simulink model "porte_avion_echantionne_model"  (R2025b)
settings: Solver=VariableStepAuto  StartTime=0.0  StopTime=100  RelTol=1e-3
values from neighbouring files (symbols this model uses):
  Ac = [0 1 0 0 ... (first row only)    [porte_avion_ech.m]
  Ad = ssd.A    [porte_avion_ech.m]
  Bc = [0 ... (first row only)    [porte_avion_ech.m]
  Bd = ssd.B    [porte_avion_ech.m]
  Cc = [0 0 1 0]    [porte_avion_ech.m]
  Cd = ssd.C    [porte_avion_ech.m]
  Hc = -1 / (Cc * ((Ac - Bc*Kc) \ Bc))    [porte_avion_ech.m]
  Hd = 1 / (Cd * ((eye(4) - (Ad - Bd*Kd)) \ Bd))    [porte_avion_ech.m]
  Kc = place(Ac, Bc, poles_c)    [porte_avion_ech.m]
  Kd = place(Ad, Bd, poles_d)    [porte_avion_ech.m]
  Ts = Tss(3)    [porte_avion_ech.m]
  X_0 = [x_0 ... (first row only)    [porte_avion_ech.m]
undefined symbols (not defined in the file or in its folder): A, A_obs, B, B_obs, C, C_obs, D, H, K, L_obs, r
settings Model: Creator=victor  LastModifiedBy=victor

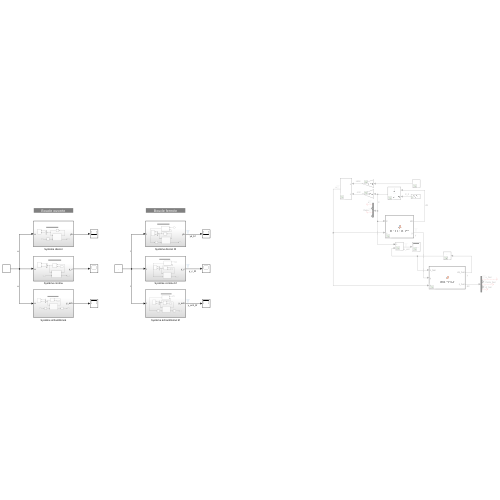
[thumbnail: Simulink's stored preview of the top-level diagram]
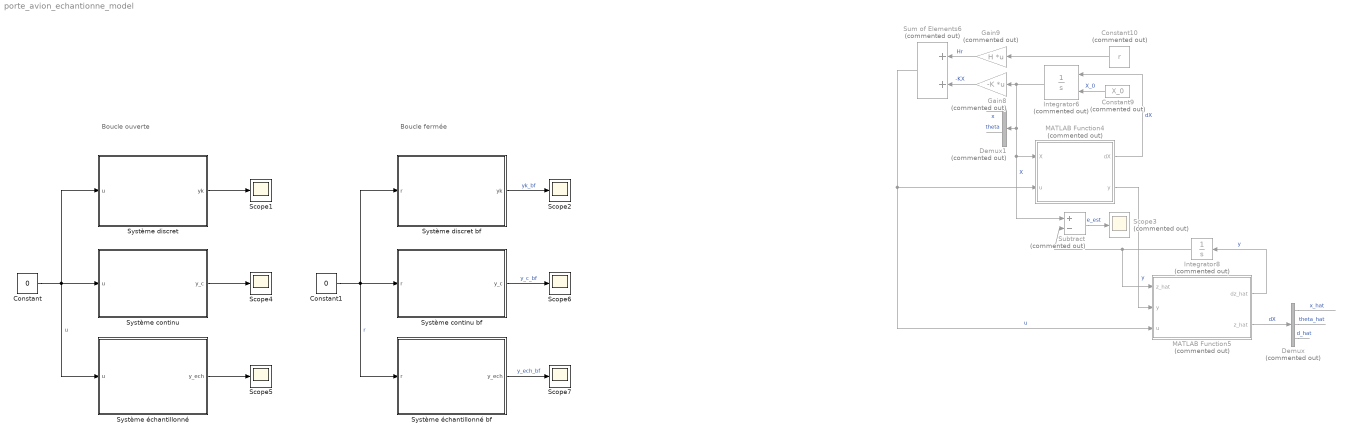
== system porte_avion_echantionne_model ==
  note: Boucle ouverte
  note: Boucle fermée
  Constant : Constant  Value=0
  Constant1 : Constant  Value=0
  Constant10 : Constant  Commented=on  Value=r
  Constant9 : Constant  Commented=on  Value=X_0
  Demux : Demux  Commented=on  Outputs=5
  Demux1 : Demux  Commented=on
  Gain8 : Gain  Commented=on  Gain=-K  Multiplication=Matrix(K*u)
  Gain9 : Gain  Commented=on  Gain=H  Multiplication=Matrix(K*u)
  Integrator6 : Integrator  Commented=on  InitialConditionSource=external
  Integrator8 : Integrator  Commented=on  InitialCondition=zeros(5, 1)
  MATLAB Function4 : MATLAB Function  Commented=on  TreatAsAtomicUnit=on
  MATLAB Function5 : MATLAB Function  Commented=on  TreatAsAtomicUnit=on
  Scope{1..2,4..7} (6 alike) : Scope
      Scope1 settings: ActiveDisplayYMinimum=-1  ActiveDisplayYMaximum=1
      Scope2 settings: ActiveDisplayYMinimum=-1  ActiveDisplayYMaximum=1  DataLoggingVariableName=ScopeData7
      Scope4 settings: ActiveDisplayYMinimum=-0.17297207419150878  ActiveDisplayYMaximum=0.36828496975347796  DataLoggingVariableName=ScopeData4
      Scope5 settings: ActiveDisplayYMinimum=-0.17297207419150878  ActiveDisplayYMaximum=0.36828496975347796  DataLoggingVariableName=ScopeData5
      Scope6 settings: ActiveDisplayYMinimum=-0.17297207419150878  ActiveDisplayYMaximum=0.36828496975347796  DataLoggingVariableName=ScopeData8
      Scope7 settings: ActiveDisplayYMinimum=-0.17297207419150878  ActiveDisplayYMaximum=0.36828496975347796  DataLoggingVariableName=ScopeData9
  Scope3 : Scope  Commented=on
      settings: ActiveDisplayYMinimum=-1.369875447599938  ActiveDisplayYMaximum=0.62027967456851218  DataLoggingVariableName=ScopeData3
  Subtract : Sum  Commented=on  Inputs=+-
  Sum of Elements6 : Sum  Commented=on
  Système continu : Subsystem
  Système continu bf : Subsystem
  Système discret : Subsystem
  Système discret bf : Subsystem
  Système échantillonné : Subsystem
  Système échantillonné bf : Subsystem
  wires:
  Demux/1 -> ?  "x_hat"
  Gain8/1 -> Sum of Elements6/2  "-KX"
  Demux/5 -> ?  "d_hat"
  Demux1/3 -> ?  "theta"
  MATLAB Function5/1(dz_hat) -> Integrator8/1  "y"
  Sum of Elements6/1 -> MATLAB Function4/2(u), MATLAB Function5/3(u)  "u"
  Demux/3 -> ?  "theta_hat"
  Integrator8/1 -> MATLAB Function5/1("z_hat "), Subtract/2
  Demux1/1 -> ?  "x"
  MATLAB Function4/2(y) -> MATLAB Function5/2(y)  "y"
  Gain9/1 -> Sum of Elements6/1  "Hr"
  MATLAB Function4/1(dX) -> Integrator6/1  "dX"
  MATLAB Function5/2(z_hat) -> Demux/1  "dX"
  Constant10/1 -> Gain9/1
  Subtract/1 -> Scope3/1  "e_est"
  Integrator6/1 -> Subtract/1, MATLAB Function4/1(X), Demux1/1, Gain8/1  "X"
  Constant9/1 -> Integrator6/2  "X_0"
  Constant/1 -> Système échantillonné/1(u), Système discret/1(u), Système continu/1(u)  "u"
  Système discret/1(yk) -> Scope1/1
  Système continu/1(y_c) -> Scope4/1
  Système échantillonné/1(y_ech) -> Scope5/1
  Système discret bf/1(yk) -> Scope2/1  "yk_bf"
  Constant1/1 -> Système échantillonné bf/1(r), Système discret bf/1(r), Système continu bf/1(r)  "r"
  Système continu bf/1(y_c) -> Scope6/1  "y_c_bf"
  Système échantillonné bf/1(y_ech) -> Scope7/1  "y_ech_bf"

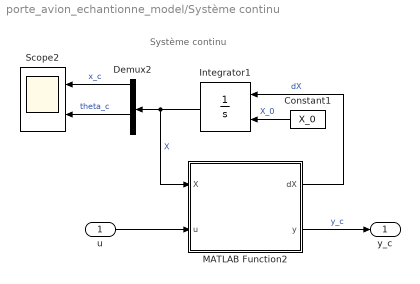
== system porte_avion_echantionne_model/Système continu ==
  note: Système continu
  u : Inport
  Constant1 : Constant  Value=X_0
  Demux2 : Demux
  Integrator1 : Integrator  InitialConditionSource=external
  MATLAB Function2 : MATLAB Function  TreatAsAtomicUnit=on
  Scope2 : Scope  NumInputPorts=2
      settings: ActiveDisplayYMinimum=-33.650451529708675  ActiveDisplayYMaximum=4.0880049092553845  DataLoggingVariableName=ScopeData2
  y_c : Outport
  wires:
  Integrator1/1 -> MATLAB Function2/1(X), Demux2/1  "X"
  Demux2/1 -> Scope2/1  "x_c"
  Demux2/3 -> Scope2/2  "theta_c"
  Constant1/1 -> Integrator1/2  "X_0"
  u/1 -> MATLAB Function2/2(u)
  MATLAB Function2/1(dX) -> Integrator1/1  "dX"
  MATLAB Function2/2(y) -> y_c/1  "y_c"

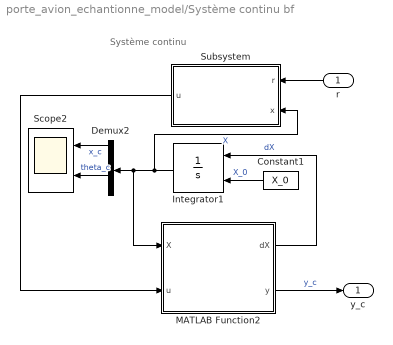
== system porte_avion_echantionne_model/Système continu bf ==
  note: Système continu
  r : Inport
  Constant1 : Constant  Value=X_0
  Demux2 : Demux
  Integrator1 : Integrator  InitialConditionSource=external
  MATLAB Function2 : MATLAB Function  TreatAsAtomicUnit=on
  Scope2 : Scope  NumInputPorts=2
      settings: ActiveDisplayYMinimum=-33.650451529708675  ActiveDisplayYMaximum=4.0880049092553845  DataLoggingVariableName=ScopeData2
  Subsystem : Subsystem
  y_c : Outport
  wires:
  Integrator1/1 -> Subsystem/2(x), MATLAB Function2/1(X), Demux2/1  "X"
  Demux2/1 -> Scope2/1  "x_c"
  Demux2/3 -> Scope2/2  "theta_c"
  Constant1/1 -> Integrator1/2  "X_0"
  Subsystem/1(u) -> MATLAB Function2/2(u)
  MATLAB Function2/1(dX) -> Integrator1/1  "dX"
  MATLAB Function2/2(y) -> y_c/1  "y_c"
  r/1 -> Subsystem/1(r)

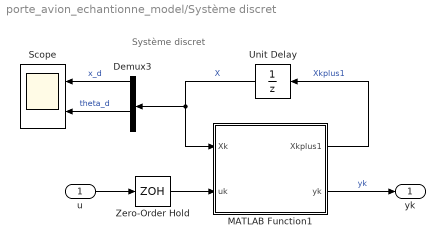
== system porte_avion_echantionne_model/Système discret ==
  note: Système discret
  u : Inport
  Demux3 : Demux
  MATLAB Function1 : MATLAB Function  TreatAsAtomicUnit=on  SystemSampleTime=Ts
  Scope : Scope  NumInputPorts=2
      settings: ActiveDisplayYMinimum=-1  ActiveDisplayYMaximum=1
  Unit Delay : UnitDelay  InitialCondition=X_0  SampleTime=-1  HasFrameUpgradeWarning=on
  Zero-Order Hold : ZeroOrderHold  SampleTime=-1
  yk : Outport
  wires:
  Demux3/1 -> Scope/1  "x_d"
  Zero-Order Hold/1 -> MATLAB Function1/2(uk)
  Unit Delay/1 -> Demux3/1, MATLAB Function1/1(Xk)  "X"
  MATLAB Function1/2(yk) -> yk/1  "yk"
  Demux3/3 -> Scope/2  "theta_d"
  MATLAB Function1/1(Xkplus1) -> Unit Delay/1  "Xkplus1"
  u/1 -> Zero-Order Hold/1

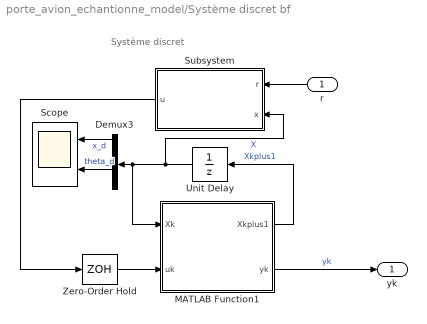
== system porte_avion_echantionne_model/Système discret bf ==
  note: Système discret
  r : Inport
  Demux3 : Demux
  MATLAB Function1 : MATLAB Function  TreatAsAtomicUnit=on  SystemSampleTime=Ts
  Scope : Scope  NumInputPorts=2
      settings: ActiveDisplayYMinimum=-1  ActiveDisplayYMaximum=1
  Subsystem : Subsystem
  Unit Delay : UnitDelay  InitialCondition=X_0  SampleTime=-1  HasFrameUpgradeWarning=on
  Zero-Order Hold : ZeroOrderHold  SampleTime=-1
  yk : Outport
  wires:
  Demux3/1 -> Scope/1  "x_d"
  Zero-Order Hold/1 -> MATLAB Function1/2(uk)
  Unit Delay/1 -> Subsystem/2(x), MATLAB Function1/1(Xk), Demux3/1  "X"
  MATLAB Function1/2(yk) -> yk/1  "yk"
  Demux3/3 -> Scope/2  "theta_d"
  MATLAB Function1/1(Xkplus1) -> Unit Delay/1  "Xkplus1"
  r/1 -> Subsystem/1(r)
  Subsystem/1(u) -> Zero-Order Hold/1

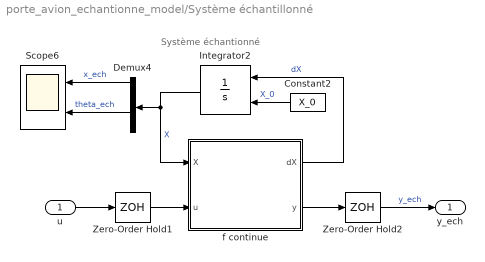
== system porte_avion_echantionne_model/Système échantillonné ==
  note: Système échantionné
  u : Inport
  Constant2 : Constant  Value=X_0
  Demux4 : Demux
  Integrator2 : Integrator  InitialConditionSource=external
  Scope6 : Scope  NumInputPorts=2
      settings: ActiveDisplayYMinimum=-33.650451529708675  ActiveDisplayYMaximum=4.0880049092553845  DataLoggingVariableName=ScopeData6
  Zero-Order Hold1 : ZeroOrderHold  SampleTime=Ts
  Zero-Order Hold2 : ZeroOrderHold  SampleTime=Ts
  f continue : MATLAB Function  TreatAsAtomicUnit=on
  y_ech : Outport
  wires:
  Constant2/1 -> Integrator2/2  "X_0"
  Zero-Order Hold1/1 -> f continue/2(u)
  Integrator2/1 -> Demux4/1, f continue/1(X)  "X"
  Demux4/1 -> Scope6/1  "x_ech"
  Demux4/3 -> Scope6/2  "theta_ech"
  f continue/1(dX) -> Integrator2/1  "dX"
  f continue/2(y) -> Zero-Order Hold2/1
  Zero-Order Hold2/1 -> y_ech/1  "y_ech"
  u/1 -> Zero-Order Hold1/1

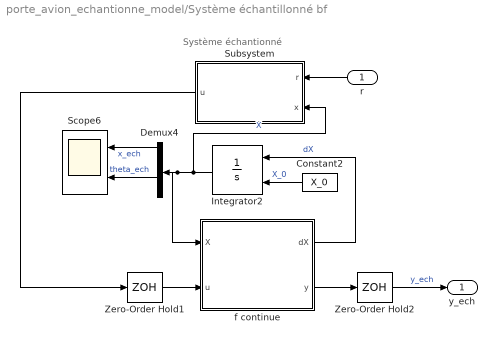
== system porte_avion_echantionne_model/Système échantillonné bf ==
  note: Système échantionné
  r : Inport
  Constant2 : Constant  Value=X_0
  Demux4 : Demux
  Integrator2 : Integrator  InitialConditionSource=external
  Scope6 : Scope  NumInputPorts=2
      settings: ActiveDisplayYMinimum=-33.650451529708675  ActiveDisplayYMaximum=4.0880049092553845  DataLoggingVariableName=ScopeData6
  Subsystem : Subsystem
  Zero-Order Hold1 : ZeroOrderHold  SampleTime=Ts
  Zero-Order Hold2 : ZeroOrderHold  SampleTime=Ts
  f continue : MATLAB Function  TreatAsAtomicUnit=on
  y_ech : Outport
  wires:
  Constant2/1 -> Integrator2/2  "X_0"
  Zero-Order Hold1/1 -> f continue/2(u)
  Integrator2/1 -> Subsystem/2(x), f continue/1(X), Demux4/1  "X"
  Demux4/1 -> Scope6/1  "x_ech"
  Demux4/3 -> Scope6/2  "theta_ech"
  f continue/1(dX) -> Integrator2/1  "dX"
  f continue/2(y) -> Zero-Order Hold2/1
  Zero-Order Hold2/1 -> y_ech/1  "y_ech"
  Subsystem/1(u) -> Zero-Order Hold1/1
  r/1 -> Subsystem/1(r)

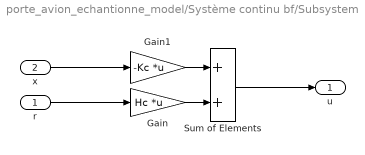
== system porte_avion_echantionne_model/Système continu bf/Subsystem ==
  r : Inport
  x : Inport  Port=2
  Gain : Gain  Gain=Hc  Multiplication=Matrix(K*u)
  Gain1 : Gain  Gain=-Kc  Multiplication=Matrix(K*u)
  Sum of Elements : Sum
  u : Outport
  wires:
  Sum of Elements/1 -> u/1
  Gain1/1 -> Sum of Elements/1
  x/1 -> Gain1/1
  Gain/1 -> Sum of Elements/2
  r/1 -> Gain/1

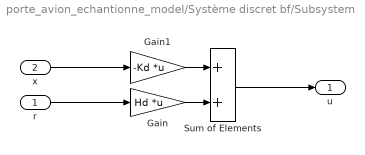
== system porte_avion_echantionne_model/Système discret bf/Subsystem ==
  r : Inport
  x : Inport  Port=2
  Gain : Gain  Gain=Hd  Multiplication=Matrix(K*u)
  Gain1 : Gain  Gain=-Kd  Multiplication=Matrix(K*u)
  Sum of Elements : Sum
  u : Outport
  wires:
  Sum of Elements/1 -> u/1
  Gain1/1 -> Sum of Elements/1
  x/1 -> Gain1/1
  Gain/1 -> Sum of Elements/2
  r/1 -> Gain/1

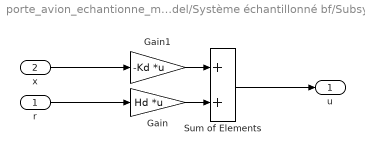
== system porte_avion_echantionne_model/Système échantillonné bf/Subsystem ==
  r : Inport
  x : Inport  Port=2
  Gain : Gain  Gain=Hd  Multiplication=Matrix(K*u)
  Gain1 : Gain  Gain=-Kd  Multiplication=Matrix(K*u)
  Sum of Elements : Sum
  u : Outport
  wires:
  Sum of Elements/1 -> u/1
  Gain1/1 -> Sum of Elements/1
  x/1 -> Gain1/1
  Gain/1 -> Sum of Elements/2
  r/1 -> Gain/1

== matlab function porte_avion_echantionne_model/Système échantillonné bf/f continue ==
  data: X input; u input; dX output; y output; Ac parameter; Bc parameter; Cc parameter
function [dX, y]= porte_avion_dyn(X, u, Ac, Bc, Cc)
dX = Ac*X + Bc*u;
y = Cc*X;
end

== matlab function porte_avion_echantionne_model/Système discret/MATLAB Function1 ==
  data: Xk input; uk input; Xkplus1 output; yk output; Ad parameter; Bd parameter; Cd parameter
function [Xkplus1, yk]= porte_avion_dyn(Xk, uk, Ad, Bd, Cd)
Xkplus1 = zeros(4, 1)
Xkplus1 = Ad*Xk + Bd*uk;
yk = Cd*Xk;
end

== matlab function porte_avion_echantionne_model/Système continu/MATLAB Function2 ==
  data: X input; u input; dX output; y output; Ac parameter; Bc parameter; Cc parameter
function [dX, y]= porte_avion_dyn(X, u, Ac, Bc, Cc)
dX = Ac*X + Bc*u;
y = Cc*X;
end

== matlab function porte_avion_echantionne_model/Système échantillonné/f continue ==
  data: X input; u input; dX output; y output; Ac parameter; Bc parameter; Cc parameter
function [dX, y]= porte_avion_dyn(X, u, Ac, Bc, Cc)
dX = Ac*X + Bc*u;
y = Cc*X;
end

== matlab function porte_avion_echantionne_model/Système continu bf/MATLAB Function2 ==
  data: X input; u input; dX output; y output; Ac parameter; Bc parameter; Cc parameter
function [dX, y]= porte_avion_dyn(X, u, Ac, Bc, Cc)
dX = Ac*X + Bc*u;
y = Cc*X;
end

== matlab function porte_avion_echantionne_model/MATLAB Function4 ==
  data: X input; u input; dX output; y output; A parameter; B parameter; C parameter; D parameter
function [dX, y]= porte_avion_dyn(X, u, A, B, C, D)
dX = A*X + B*u;
y = C2*X + D2*u;
end

== matlab function porte_avion_echantionne_model/MATLAB Function5 ==
  data: dz_hat output; z_hat input; y input; u input; A_obs parameter; z_hat output; B_obs parameter; C_obs parameter; L_obs parameter
function [dz_hat, z_hat]= observateur(z_hat, y, u, A_obs, B_obs, C_obs, L_obs)
dz_hat = zeros(5, 1);
dz_hat = A_obs*z_hat + B_obs*u + L_obs*(y - C_obs*z_hat);
end

== matlab function porte_avion_echantionne_model/Système discret bf/MATLAB Function1 ==
  data: Xk input; uk input; Xkplus1 output; yk output; Ad parameter; Bd parameter; Cd parameter
function [Xkplus1, yk]= porte_avion_dyn(Xk, uk, Ad, Bd, Cd)
Xkplus1 = zeros(4, 1)
Xkplus1 = Ad*Xk + Bd*uk;
yk = Cd*Xk;
end
